simulink model "canonicalWalking"  (R2014a)
settings: Solver=FixedStepDiscrete  StartTime=0.0  StopTime=inf  FixedStep=sample_time  RelTol=1e-3
libraries: slrtlib x3
settings Model: SimulationMode=external  BufferReuse=off  Creator=wmartin  LastModifiedBy=drl
settings SolverCC: EnableConcurrentExecution=on
settings DataIOCC: MaxDataPoints=1000000000  SaveFormat=StructureWithTime  SaveOutput=off  SaveTime=off
settings OptimizationCC: BlockReduction=off  OptimizeBlockIOStorage=off  BufferReuse=off  GlobalBufferReuse=off  ExpressionFolding=off  ExpressionDepthLimit=2147483647  LocalBlockOutputs=off  SimCompilerOptimization=On
settings DebuggingCC: UnderspecifiedInitializationDetection=Classic  StateNameClashWarn=warning
settings HardwareCC: ProdIntDivRoundTo=Zero  ProdEndianess=LittleEndian  ProdHWDeviceType=Generic->32-bit x86 compatible
settings ModelReferenceCC: UpdateModelReferenceTargets=IfOutOfDate  ModelReferenceNumInstancesAllowed=Single  ModelReferenceMinAlgLoopOccurrences=on
settings RTWCC: SystemTargetFile=slrt.tlc  TemplateMakefile=slrt_default_tmf  Description=Simulink Real-Time  RTWVerbose=off  ProcessScript=slrt_make_rtw_hook  RTWCompilerOptimization=On
settings SimulinkRealTimeCC: GeneratePreprocessorConditionals=Disable all  EnableShiftOperators=on  RL32LogBufSizeModifier=100000000

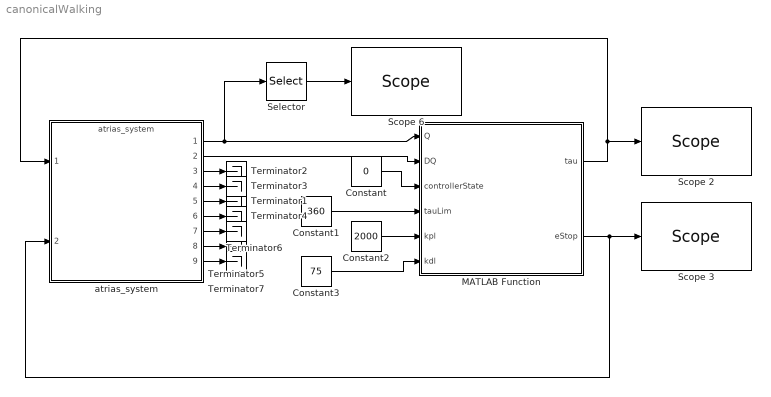
== system canonicalWalking ==
  Constant : Constant  Value=0
  Constant1 : Constant  Value=360
  Constant2 : Constant  Value=2000
  Constant3 : Constant  Value=75
  MATLAB Function : MATLAB Function  TreatAsAtomicUnit=on
  Scope 2 : slrtlib/Displays and Logging/Scope   scopeno=2  scopetype=Target  autostart=on  viewmode=Numerical  formatstr='%15.6f'  grid=on  ylimits=[0,0]  nosamples=100  noprepostsamples=0  interleave=1  triggermode=FreeRun  triggersignal=1  trigsignalfromport=off  triggerlevel=0.0  triggerslope=Either  triggerscope=1  triggersample=0  filename=data.dat  mode=Lazy  writesize=512  autorestart=off  dynamicfilemode=off  maxwritefilesize=512*1024^2
  Scope 3 : slrtlib/Displays and Logging/Scope   scopeno=3  scopetype=Target  autostart=on  viewmode=Numerical  formatstr='%15.6f'  grid=on  ylimits=[0,0]  nosamples=100  noprepostsamples=0  interleave=1  triggermode=FreeRun  triggersignal=1  trigsignalfromport=off  triggerlevel=0.0  triggerslope=Either  triggerscope=1  triggersample=0  filename=data.dat  mode=Lazy  writesize=512  autorestart=off  dynamicfilemode=off  maxwritefilesize=512*1024^2
  Scope 6 : slrtlib/Displays and Logging/Scope   scopeno=6  scopetype=Target  autostart=on  viewmode=Numerical  formatstr='%15.6f'  grid=on  ylimits=[0,0]  nosamples=100  noprepostsamples=0  interleave=1  triggermode=FreeRun  triggersignal=1  trigsignalfromport=off  triggerlevel=0.0  triggerslope=Either  triggerscope=1  triggersample=0  filename=data.dat  mode=Lazy  writesize=512  autorestart=off  dynamicfilemode=off  maxwritefilesize=512*1024^2
  Selector : Selector  InputPortWidth=13  Indices=[11:13]
  Terminator{1..7} (7 alike) : Terminator
  atrias_system : ModelReference  ModelNameDialog=atrias_system  SimulationMode=Normal  ModelReferenceVersion=1.1786  CopyOfModelName=atrias_system  DefaultDataLogging=on
  wires:
  atrias_system/2 -> MATLAB Function/2(DQ)
  MATLAB Function/1(tau) -> atrias_system/1, Scope 2/1
  MATLAB Function/2(eStop) -> atrias_system/2, Scope 3/1
  atrias_system/3 -> Terminator2/1
  atrias_system/4 -> Terminator3/1
  atrias_system/5 -> Terminator1/1
  atrias_system/6 -> Terminator4/1
  Constant/1 -> MATLAB Function/3(controllerState)
  atrias_system/1 -> Selector/1, MATLAB Function/1(Q)
  Selector/1 -> Scope 6/1
  Constant1/1 -> MATLAB Function/4(tauLim)
  atrias_system/8 -> Terminator5/1
  atrias_system/7 -> Terminator6/1
  atrias_system/9 -> Terminator7/1
  Constant2/1 -> MATLAB Function/5(kpl)
  Constant3/1 -> MATLAB Function/6(kdl)

== matlab function canonicalWalking/MATLAB Function ==
  data: Q input; tau output; DQ input; controllerState input; eStop output; tauLim input; kpl input; kdl input
function [tau, eStop] = canonicalWalking(Q, DQ, controllerState, tauLim, kpl, kdl)
%CANONICALWALKING Canonical walking controller used in HSCC 2014 paper.
%
% Description:
%   This controller implements a variation of hybrid zero dynamics on the
%		planar model of ATRIAS. This is the same controller (transcribed to 
%		Simulink) used in the 2014 HSCC paper.
%
% Notes:
% 	- State indexes (rBl rBm rAl rAm lBl lBm lAl lAm rHm lHm bR bY bP) 
%   - Input indexes (rB rA rH lB lA lH)
%
% TODO:
%   - Find units of tau and set limits
%   - Enable ds computation, xa0dot computation and leg switching
%   - Use hip controller that applies zero knee force

    right = 0;
    left = 1;

    % TEMPORARY HIP BUG 1 rev off
    Q(9) = Q(9) + 2*pi;
    
    % Initialize variable
    persistent stanceLeg;
    if isempty(stanceLeg); stanceLeg = left; end;
    eStop = false;
    
	% Optimized gait parameters
	A_OPT = [3.13058278616339, 3.38621285654106, 2.26312258300192, 3.72562917760651, 2.21768467271887, 3.00343594477559, 2.63518033870867;
		3.88033369474228, 3.81628375091666, 3.64791062079225, 3.54302625758800, 3.60125936599999, 3.45364342671221, 3.37022239691970;
		2.63529972490620, 2.22706769173603, 3.56813326557356, 0.695310365268170, 2.91237158193484, 2.90041027511901, 3.13100976580989;
		3.37031174388957, 3.27783500873126, 2.93958409614047, 3.48644831132767, 4.39294714621698, 3.93787692520441, 3.88009422366450];
	D_OPT = [1.53378042226602, -6.73854164123482, 8.77503956762755, -9.04766702932585, 4.71450763234033, -2.20953363640152;
		-0.384299662953726, -1.01023878074645, -0.629306179225527, 0.349398650471944, -0.885695635726687, -0.500526178755031;
		-2.44939219902102, 8.04639344302521, -17.2369374018324, 13.3023673000000, -0.0717678408949780, 1.38359694414531;
		-0.554860410949804, -2.02950547554476, 3.28118529112322, 5.43899300933585, -2.73042132607544, -0.346696209239457];
	X_OPT = [2.63529972490620; 3.37031174388957; 3.13058278616339; 3.88033369474228];
	P_OPT = [-0.286373623667230, 0.177718855319307].';
    
    % Define actuator gains
    kph = 1500; kdh = 10;
    
    % Initialize input vector to zeros
    u = zeros(6,1);
    
	% Compute hip actuator torques using PD controller
	u([3 6]) = (0 - Q([9 10]))*kph + (0 - DQ([9 10]))*kdh;
    
    % Main controller state machine
    switch controllerState
        case 0
            % Compute leg actuator torques using PD controller
            u([2 1 5 4]) = (X_OPT - Q([4 2 8 6]))*kpl + (0 - DQ([4 2 8 6]))*kdl;
            
        case 1
            % Grab desired actuator states
            switch stanceLeg
                case left
                    xa = [Q([11 7 5 3 1 9 10]); DQ([11 7 5 3 1 9 10])];
                case right
                    xa = [Q([11 3 1 7 5 10 9]); DQ([11 3 1 7 5 10 9])];
                otherwise; eStop = true; xa = zeros(14,1);
            end % switch

            % Compute time invariant parameter
            s = -((xa(1) + (xa(2) + xa(3))/2) + P_OPT(1) - pi)/(P_OPT(2) - P_OPT(1));
            ds = -(xa(8) + (xa(9) + xa(10))/2)/(P_OPT(2) - P_OPT(1));
            
            % Bound time invariant parameter between 0 and 1 (or close to it)
            s = clamp(s, -0.001, 1);
            ds = clamp(ds, 0, inf);
            
            % Compute desired outputs
            xa0 = A_OPT(:,1)*(1-s)^6 + 6*A_OPT(:,2)*s*(1-s)^5 + ...
                15*A_OPT(:,3)*s^2*(1-s)^4 + 20*A_OPT(:,4)*s^3*(1-s)^3 + ...
                15*A_OPT(:,5)*s^4*(1-s)^2 + 6*A_OPT(:,6)*s^5*(1-s) + A_OPT(:,7)*s^6;
%             xa0dot = D_OPT(:,1)*(1-s)^5 + 5*D_OPT(:,2)*s*(1-s)^4 + ...
%                 10*D_OPT(:,3)*s^2*(1-s)^3 + 10*D_OPT(:,4)*s^3*(1-s)^2 + ...
%                 5*D_OPT(:,5)*s^4*(1-s) + D_OPT(:,6)*s^5;
            xa0dot = ds; % TODO: Remove once working
            
            % Compute actuator torques using PD controller
            switch stanceLeg
                case left
                    u([5 4 2 1]) = (xa0 - Q([8 6 4 2]))*kpl + (xa0dot - DQ([8 6 4 2]))*kdl;
                case right
                    u([2 1 5 4]) = (xa0 - Q([4 2 8 6]))*kpl + (xa0dot - DQ([4 2 8 6]))*kdl;
            end % switch
            
            % Determine when to switch stance legs
            if s > 0.98
                % Check which leg is the stance leg
                switch stanceLeg
                    case left; stanceLeg = right;
                    case right; stanceLeg = left;
                end % switch
            end % if
            
        case 2
            % Compute leg actuator torques using virtual damper
            u = (0 - DQ([4 2 9 8 6 10])).*[kpl kpl kdl kpl kpl kdl].';
        otherwise; eStop = true;
    end % switch
    
    % Limit torques to be cautious
	tau = clamp(u, -tauLim, tauLim);

end % canonicalWalking

function b = clamp(a, lim1, lim2)
%CLAMP Clamp value between two values.
	
	% Find which limit is min and max
	aMin = min(lim1);
	aMax = max(lim2);

	% Clamp value between limits
	b = max(min(a, aMax), aMin);
end % clamp
